simulink model "connect_pend_PD"  (R2019b)
settings: Solver=VariableStepAuto  StartTime=0.0  StopTime=10.0  RelTol=1e-3
values from neighbouring files (symbols this model uses):
  dampener = 100    [anujay_single_pendulum_same.m]    (also in connect_pend.m; connect_pend_runner.m = 1; double_pend_setup.m = [50, 0; 0, 50])
  Dm1 = 30    [anujay_single_pendulum_same.m]    (also in connect_pend.m; connect_pend_runner.m; double_pend_setup.m = [30,0;0,30])
  Dm2 = 20    [connect_pend_runner.m]
  g = 9.81    [G.m]    (also in connect_pend_runner.m; run.m; single_pend_runner.m = -9.81)
  Km1 = 30    [anujay_single_pendulum_same.m]    (also in connect_pend.m; connect_pend_runner.m; double_pend_setup.m = [30, 0; 0 30])
  Km2 = 20    [connect_pend_runner.m]
  l1 = 1.0    (= 1)    [connect_pend.m]    (also in connect_pend_runner.m)
  l2 = l1    (= 1)    [connect_pend_runner.m]    (also in single_pend_runner.m = 3)
  m1 = 1.0    (= 1)    [connect_pend.m]    (also in connect_pend_runner.m)
  m2 = 1.0 + m1    (= 2)    [connect_pend.m]    (also in connect_pend_runner.m; single_pend_runner.m = 10)
  spring = 100    [anujay_single_pendulum_same.m]    (also in connect_pend.m; connect_pend_runner.m = 10; double_pend_setup.m = [50, 0; 0, 50])
libraries: robotcorelib x1
settings Model: Creator=nathanielgoldfarb  LastModifiedBy=nathanielgoldfarb

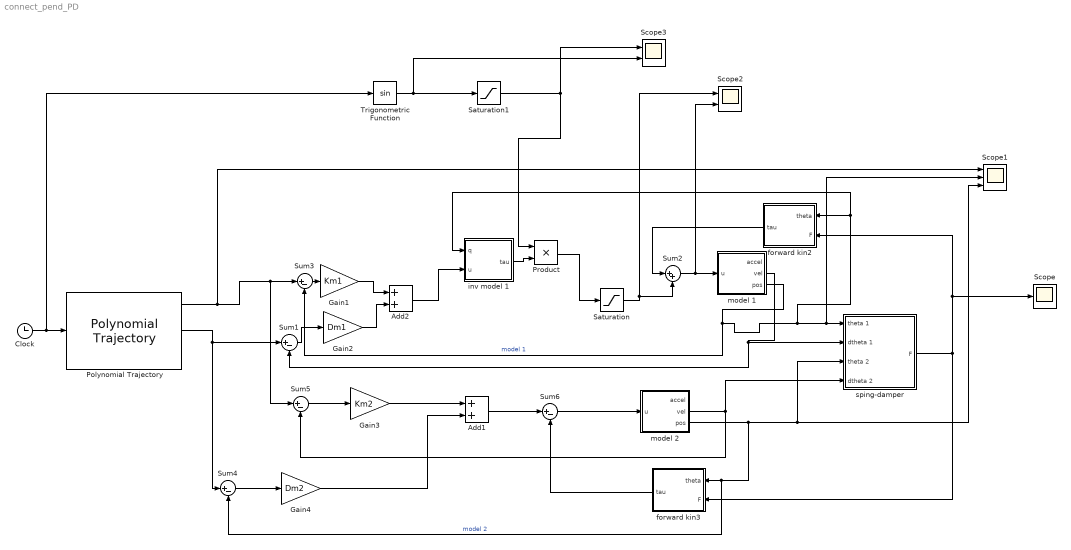
== system connect_pend_PD ==
  Add1 : Sum
  Add2 : Sum
  Clock : Clock
  Gain1 : Gain  Gain=Km1
  Gain2 : Gain  Gain=Dm1
  Gain3 : Gain  Gain=Km2
  Gain4 : Gain  Gain=Dm2
  Polynomial Trajectory : robotcorelib/Polynomial Trajectory  WaypointSource=Internal  Waypoints=[ -pi , 0 ]  TimePoints=[ 0, 3]  TimeInterval=[ 1, 4 ]  Method=Cubic Polynomial  ParameterSource=Internal  VelocityBoundaryCondition=zeros( 1, 2 )  AccelerationBoundaryCondition=zeros( 2, 5 )  SimulateUsing=Interpreted execution
      settings: SourceProductName=Robotics System Toolbox  SourceProductBaseCode=RO
  Product : Product
  Saturation : Saturate  UpperLimit=1  LowerLimit=-1
  Saturation1 : Saturate  UpperLimit=1  LowerLimit=0
  Scope : Scope
  Scope1 : Scope  NumInputPorts=3
  Scope2 : Scope  NumInputPorts=2
  Scope3 : Scope  NumInputPorts=2
  Sum{1,3..6} (5 alike) : Sum  Inputs=|+-
  Sum2 : Sum  Inputs=|++
  Trigonometric Function : Trigonometry
  forward kin2 : Subsystem
  forward kin3 : Subsystem
  inv model 1 : Subsystem
  model 1 : Subsystem
  model 2 : Subsystem
  sping-damper : Subsystem
  wires:
  Sum1/1 -> Gain2/1
  Add2/1 -> inv model 1/2("u ")
  Gain1/1 -> Add2/1
  Gain2/1 -> Add2/2
  sping-damper/1(F) -> forward kin3/2(F), Scope/1, forward kin2/2(F)
  model 1/2(vel) -> Sum1/2, sping-damper/2(dtheta 1)
  model 2/3(pos) -> Sum4/2, forward kin3/1("theta "), Scope1/3, sping-damper/3(theta 2)  "model 2"
  model 2/2(vel) -> Sum5/2, sping-damper/4(dtheta 2)
  Clock/1 -> Trigonometric Function/1, Polynomial Trajectory/1
  Sum3/1 -> Gain1/1
  Polynomial Trajectory/1 -> Scope1/1, Sum5/1, Sum3/1
  Polynomial Trajectory/2 -> Sum4/1, Sum1/1
  Sum4/1 -> Gain4/1
  Sum5/1 -> Gain3/1
  Gain3/1 -> Add1/1
  Gain4/1 -> Add1/2
  Add1/1 -> Sum6/1
  Sum6/1 -> model 2/1("u ")
  forward kin3/1("tau ") -> Sum6/2
  model 1/3(pos) -> inv model 1/1(q), forward kin2/1("theta "), Scope1/2, sping-damper/1(theta 1), Sum3/2  "model 1"
  forward kin2/1("tau ") -> Sum2/1
  inv model 1/1("tau ") -> Product/2
  Product/1 -> Saturation/1
  Saturation/1 -> Scope2/1, Sum2/2
  Sum2/1 -> Scope2/2, model 1/1("u ")
  Trigonometric Function/1 -> Saturation1/1, Scope3/2
  Saturation1/1 -> Product/1, Scope3/1

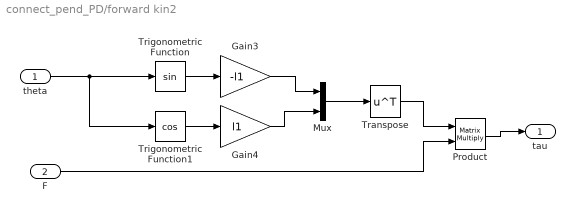
== system connect_pend_PD/forward kin2 ==
  "theta " : Inport
  F : Inport  Port=2
  Gain3 : Gain  Gain=-l1
  Gain4 : Gain  Gain=l1
  Mux : Mux  Inputs=2
  Product : Product  Multiplication=Matrix(*)
  Transpose : Math  Operator=transpose  SignedPower=off  SaturateOnIntegerOverflow=on
  Trigonometric Function : Trigonometry
  Trigonometric Function1 : Trigonometry  Operator=cos
  "tau " : Outport
  wires:
  "theta "/1 -> Trigonometric Function1/1, Trigonometric Function/1
  Gain4/1 -> Mux/2
  Trigonometric Function/1 -> Gain3/1
  Gain3/1 -> Mux/1
  Trigonometric Function1/1 -> Gain4/1
  Mux/1 -> Transpose/1
  Transpose/1 -> Product/1
  F/1 -> Product/2
  Product/1 -> "tau "/1

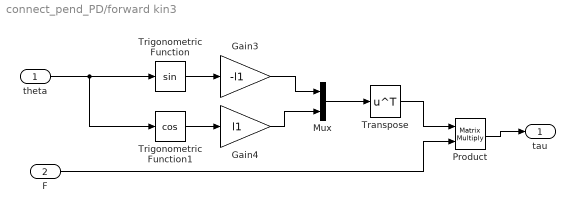
== system connect_pend_PD/forward kin3 ==
  "theta " : Inport
  F : Inport  Port=2
  Gain3 : Gain  Gain=-l1
  Gain4 : Gain  Gain=l1
  Mux : Mux  Inputs=2
  Product : Product  Multiplication=Matrix(*)
  Transpose : Math  Operator=transpose  SignedPower=off  SaturateOnIntegerOverflow=on
  Trigonometric Function : Trigonometry
  Trigonometric Function1 : Trigonometry  Operator=cos
  "tau " : Outport
  wires:
  "theta "/1 -> Trigonometric Function1/1, Trigonometric Function/1
  Gain4/1 -> Mux/2
  Trigonometric Function/1 -> Gain3/1
  Gain3/1 -> Mux/1
  Trigonometric Function1/1 -> Gain4/1
  Mux/1 -> Transpose/1
  Transpose/1 -> Product/1
  F/1 -> Product/2
  Product/1 -> "tau "/1

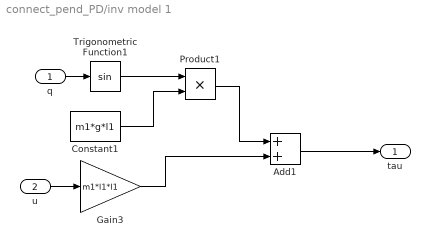
== system connect_pend_PD/inv model 1 ==
  q : Inport
  "u " : Inport  Port=2
  Add1 : Sum
  Constant1 : Constant  Value=m1*g*l1
  Gain3 : Gain  Gain=m1*l1*l1
  Product1 : Product
  Trigonometric Function1 : Trigonometry
  "tau " : Outport
  wires:
  Product1/1 -> Add1/1
  Constant1/1 -> Product1/2
  Add1/1 -> "tau "/1
  Gain3/1 -> Add1/2
  "u "/1 -> Gain3/1
  Trigonometric Function1/1 -> Product1/1
  q/1 -> Trigonometric Function1/1

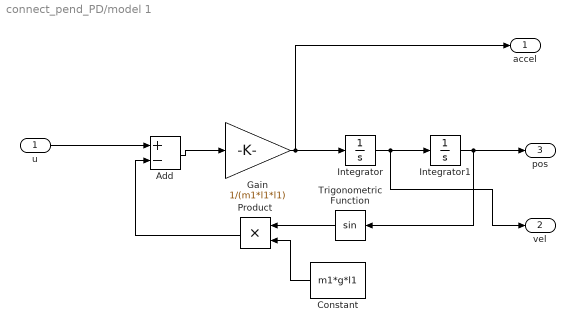
== system connect_pend_PD/model 1 ==
  "u " : Inport
  Add : Sum  Inputs=+-
  Constant : Constant  Value=m1*g*l1
  Gain : Gain  Gain=1/(m1*l1*l1)
  Integrator : Integrator
  Integrator1 : Integrator  InitialCondition=-pi
  Product : Product
  Trigonometric Function : Trigonometry
  accel : Outport
  vel : Outport  Port=2
  pos : Outport  Port=3
  wires:
  Integrator1/1 -> pos/1, Trigonometric Function/1
  "u "/1 -> Add/1
  Constant/1 -> Product/2
  Add/1 -> Gain/1
  Trigonometric Function/1 -> Product/1
  Product/1 -> Add/2
  Gain/1 -> accel/1, Integrator/1
  Integrator/1 -> vel/1, Integrator1/1

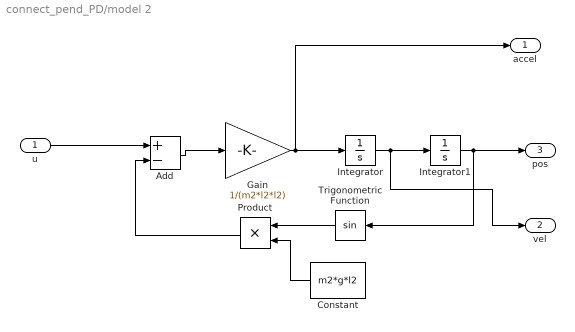
== system connect_pend_PD/model 2 ==
  "u " : Inport
  Add : Sum  Inputs=+-
  Constant : Constant  Value=m2*g*l2
  Gain : Gain  Gain=1/(m2*l2*l2)
  Integrator : Integrator
  Integrator1 : Integrator  InitialCondition=-pi
  Product : Product
  Trigonometric Function : Trigonometry
  accel : Outport
  vel : Outport  Port=2
  pos : Outport  Port=3
  wires:
  Integrator1/1 -> pos/1, Trigonometric Function/1
  "u "/1 -> Add/1
  Constant/1 -> Product/2
  Add/1 -> Gain/1
  Trigonometric Function/1 -> Product/1
  Product/1 -> Add/2
  Gain/1 -> accel/1, Integrator/1
  Integrator/1 -> vel/1, Integrator1/1

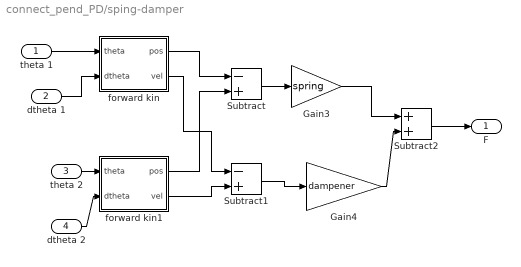
== system connect_pend_PD/sping-damper ==
  theta 1 : Inport
  dtheta 1 : Inport  Port=2
  theta 2 : Inport  Port=3
  dtheta 2 : Inport  Port=4
  Gain3 : Gain  Gain=spring
  Gain4 : Gain  Gain=dampener
  Subtract : Sum  Inputs=-+
  Subtract1 : Sum  Inputs=-+
  Subtract2 : Sum
  forward kin : Subsystem
  forward kin1 : Subsystem
  F : Outport
  wires:
  Subtract2/1 -> F/1
  forward kin/2(vel) -> Subtract1/1
  Gain4/1 -> Subtract2/2
  Subtract1/1 -> Gain4/1
  dtheta 1/1 -> forward kin/2("dtheta ")
  forward kin1/1(pos) -> Subtract/2
  theta 1/1 -> forward kin/1("theta ")
  Subtract/1 -> Gain3/1
  forward kin/1(pos) -> Subtract/1
  dtheta 2/1 -> forward kin1/2("dtheta ")
  theta 2/1 -> forward kin1/1("theta ")
  forward kin1/2(vel) -> Subtract1/2
  Gain3/1 -> Subtract2/1

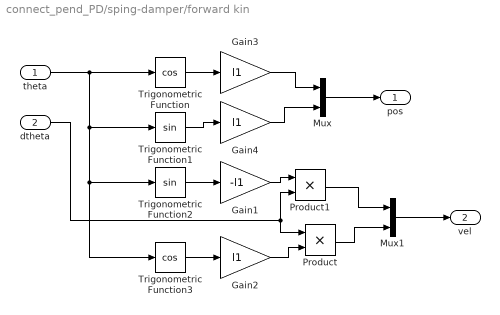
== system connect_pend_PD/sping-damper/forward kin ==
  "theta " : Inport
  "dtheta " : Inport  Port=2
  Gain1 : Gain  Gain=-l1
  Gain2 : Gain  Gain=l1
  Gain3 : Gain  Gain=l1
  Gain4 : Gain  Gain=l1
  Mux : Mux  Inputs=2
  Mux1 : Mux  Inputs=2
  Product : Product
  Product1 : Product
  Trigonometric Function : Trigonometry  Operator=cos
  Trigonometric Function1 : Trigonometry
  Trigonometric Function2 : Trigonometry
  Trigonometric Function3 : Trigonometry  Operator=cos
  pos : Outport
  vel : Outport  Port=2
  wires:
  "theta "/1 -> Trigonometric Function3/1, Trigonometric Function2/1, Trigonometric Function1/1, Trigonometric Function/1
  Gain4/1 -> Mux/2
  Trigonometric Function/1 -> Gain3/1
  Gain3/1 -> Mux/1
  Trigonometric Function1/1 -> Gain4/1
  Trigonometric Function3/1 -> Gain2/1
  Trigonometric Function2/1 -> Gain1/1
  Gain1/1 -> Product1/1
  "dtheta "/1 -> Product1/2, Product/1
  Gain2/1 -> Product/2
  Product1/1 -> Mux1/1
  Product/1 -> Mux1/2
  Mux/1 -> pos/1
  Mux1/1 -> vel/1

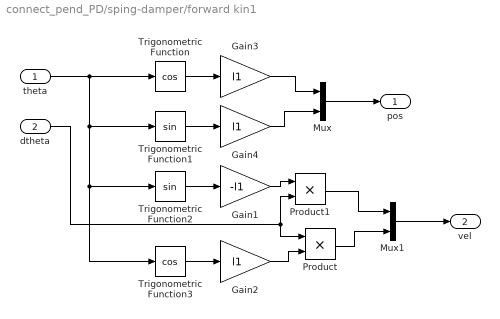
== system connect_pend_PD/sping-damper/forward kin1 ==
  "theta " : Inport
  "dtheta " : Inport  Port=2
  Gain1 : Gain  Gain=-l1
  Gain2 : Gain  Gain=l1
  Gain3 : Gain  Gain=l1
  Gain4 : Gain  Gain=l1
  Mux : Mux  Inputs=2
  Mux1 : Mux  Inputs=2
  Product : Product
  Product1 : Product
  Trigonometric Function : Trigonometry  Operator=cos
  Trigonometric Function1 : Trigonometry
  Trigonometric Function2 : Trigonometry
  Trigonometric Function3 : Trigonometry  Operator=cos
  pos : Outport
  vel : Outport  Port=2
  wires:
  "theta "/1 -> Trigonometric Function3/1, Trigonometric Function2/1, Trigonometric Function1/1, Trigonometric Function/1
  Gain4/1 -> Mux/2
  Trigonometric Function/1 -> Gain3/1
  Gain3/1 -> Mux/1
  Trigonometric Function1/1 -> Gain4/1
  Trigonometric Function3/1 -> Gain2/1
  Trigonometric Function2/1 -> Gain1/1
  Gain1/1 -> Product1/1
  "dtheta "/1 -> Product1/2, Product/1
  Gain2/1 -> Product/2
  Product1/1 -> Mux1/1
  Product/1 -> Mux1/2
  Mux/1 -> pos/1
  Mux1/1 -> vel/1
